simulink model "RespiratorSupervisor"  (R2018b)
settings: Solver=FixedStepDiscrete  StartTime=0.0  StopTime=10.0  FixedStep=MdlTS  RelTol=1e-3  EnableMultiTasking=on
libraries: LIB_AirVolumeProcessing x1, LIB_RespiratorSupervisor x1, LIB_Warning x1
settings Model: DataDictionary=RespiratorControlData.sldd  Creator=BRAUL  LastModifiedBy=VITIE
settings OptimizationCC: DefaultUnderspecifiedDataType=single  EnhancedBackFolding=on  PassReuseOutputArgsAs=Individual arguments  MaxStackSize=64  OptimizeBlockOrder=speed  DifferentSizesBufferReuse=on  OptimizationCustomize=off
settings DebuggingCC: MergeDetectMultiDrivingBlocksExec=none  ParameterTunabilityLossMsg=error
settings HardwareCC: ProdBitPerPointer=32  ProdBitPerSizeT=32  ProdBitPerPtrDiffT=32  ProdLargestAtomicInteger=Long  ProdLargestAtomicFloat=Double  ProdWordSize=32  ProdHWDeviceType=ARM Compatible->ARM Cortex
settings ModelReferenceCC: PropagateSignalLabelsOutOfModel=off
settings SFSimCC: MATLABDynamicMemAlloc=off
settings RTWCC: SystemTargetFile=ert.tlc  HardwareBoard=STM32 Nucleo F411RE  TemplateMakefile=ert_default_tmf  GenerateReport=on  Toolchain=GNU Tools for ARM Embedded Processors  BuildConfiguration=Faster Runs  IncludeHyperlinkInReport=on  LaunchReport=on  GenerateTraceInfo=on  GenerateTraceReport=on  GenerateTraceReportSl=on  GenerateTraceReportSf=on  GenerateTraceReportEml=on
settings CodeAppCC: ForceParamTrailComments=on  IgnoreCustomStorageClasses=off  OperatorAnnotations=on  SimulinkDataObjDesc=on  SFDataObjDesc=on  InsertBlockDesc=on

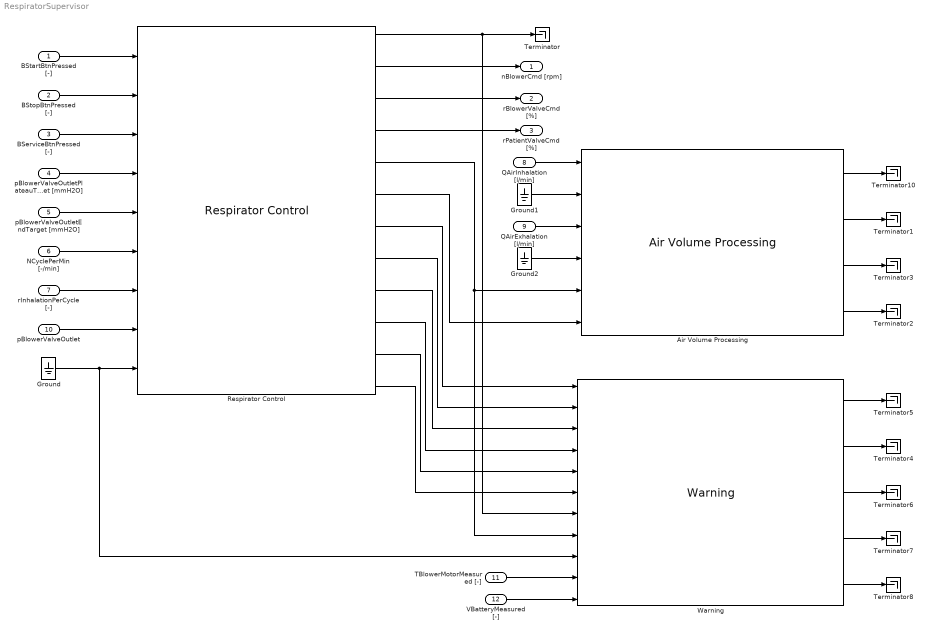
== system RespiratorSupervisor ==
  BStartBtnPressed [-] : Inport  OutDataTypeStr=boolean
  BStopBtnPressed [-] : Inport  Port=2  OutDataTypeStr=boolean
  BServiceBtnPressed [-] : Inport  Port=3  OutDataTypeStr=boolean
  pBlowerValveOutletPlateauTarget [mmH2O] : Inport  Port=4  OutDataTypeStr=single
  pBlowerValveOutletEndTarget [mmH2O] : Inport  Port=5  OutDataTypeStr=single
  NCyclePerMin [-/min] : Inport  Port=6  OutDataTypeStr=single
  rInhalationPerCycle [-] : Inport  Port=7  OutDataTypeStr=single
  QAirInhalation [l/min] : Inport  Port=8
  QAirExhalation [l/min] : Inport  Port=9
  pBlowerValveOutlet : Inport  Port=10  OutDataTypeStr=single
  TBlowerMotorMeasured [-] : Inport  Port=11
  VBatteryMeasured [-] : Inport  Port=12
  Air Volume Processing : LIB_AirVolumeProcessing/Air Volume Processing  SystemSampleTime=-1
      settings: AttributesFormatString=%<ReferenceBlock>
  Ground : Ground
  Ground1 : Ground
  Ground2 : Ground
  Respirator Control : LIB_RespiratorSupervisor/Respirator Control  SystemSampleTime=-1
      settings: AttributesFormatString=%<ReferenceBlock>
  Terminator{,1..8,10} (10 alike) : Terminator
  Warning : LIB_Warning/Warning  SystemSampleTime=-1
      settings: AttributesFormatString=%<ReferenceBlock>
  nBlowerCmd [rpm] : Outport  OutDataTypeStr=single
  rBlowerValveCmd [%] : Outport  Port=2  OutDataTypeStr=single
  rPatientValveCmd [%] : Outport  Port=3  OutDataTypeStr=single
  wires:
  BStartBtnPressed [-]/1 -> Respirator Control/1
  BStopBtnPressed [-]/1 -> Respirator Control/2
  BServiceBtnPressed [-]/1 -> Respirator Control/3
  pBlowerValveOutletPlateauTarget [mmH2O]/1 -> Respirator Control/4
  pBlowerValveOutletEndTarget [mmH2O]/1 -> Respirator Control/5
  NCyclePerMin [-/min]/1 -> Respirator Control/6
  rInhalationPerCycle [-]/1 -> Respirator Control/7
  Respirator Control/2 -> nBlowerCmd [rpm]/1
  Respirator Control/3 -> rBlowerValveCmd [%]/1
  Respirator Control/4 -> rPatientValveCmd [%]/1
  Ground/1 -> Warning/9, Respirator Control/9
  pBlowerValveOutlet/1 -> Respirator Control/8
  Respirator Control/6 -> Air Volume Processing/6
  Air Volume Processing/1 -> Terminator10/1
  Air Volume Processing/2 -> Terminator1/1
  Air Volume Processing/4 -> Terminator2/1
  Air Volume Processing/3 -> Terminator3/1
  Respirator Control/1 -> Terminator/1, Warning/7
  TBlowerMotorMeasured [-]/1 -> Warning/10
  VBatteryMeasured [-]/1 -> Warning/11
  Warning/1 -> Terminator5/1
  Warning/2 -> Terminator4/1
  Warning/3 -> Terminator6/1
  Warning/4 -> Terminator7/1
  Warning/5 -> Terminator8/1
  QAirInhalation [l/min]/1 -> Air Volume Processing/1
  QAirExhalation [l/min]/1 -> Air Volume Processing/3
  Ground1/1 -> Air Volume Processing/2
  Ground2/1 -> Air Volume Processing/4
  Respirator Control/7 -> Warning/1
  Respirator Control/8 -> Warning/2
  Respirator Control/9 -> Warning/3
  Respirator Control/10 -> Warning/4
  Respirator Control/11 -> Warning/5
  Respirator Control/12 -> Warning/6
  Respirator Control/5 -> Air Volume Processing/5, Warning/8
